simulink library "INT_CoETS_TrqCalc"  (R2016b)
settings: Solver=VariableStepAuto  StartTime=0.0  StopTime=10.0  RelTol=1e-3
settings Model: Creator=xuxingpei  LastModifiedBy=xuxingpei

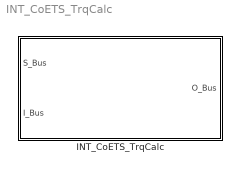
== system INT_CoETS_TrqCalc ==
  INT_CoETS_TrqCalc : Subsystem

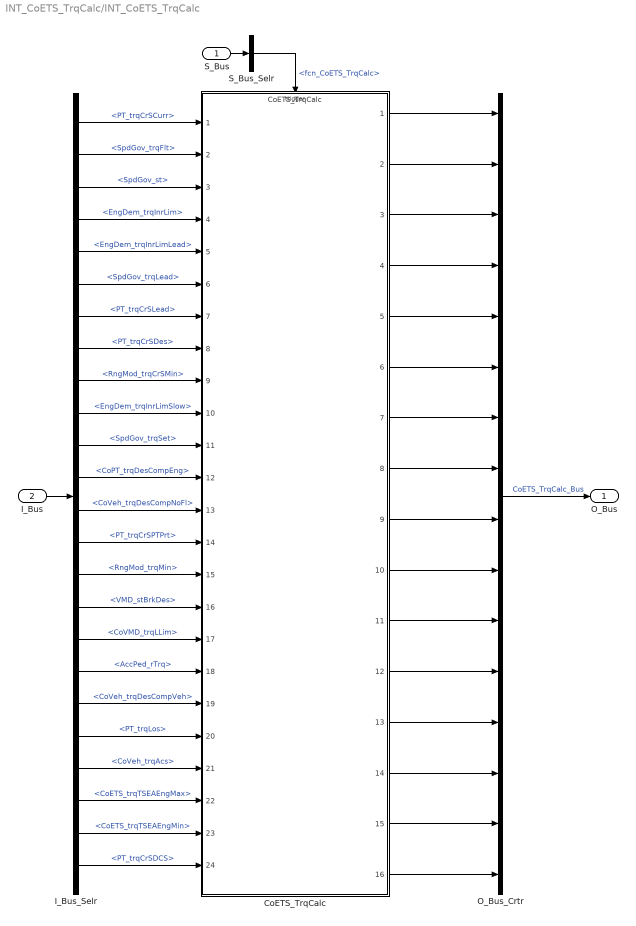
== system INT_CoETS_TrqCalc/INT_CoETS_TrqCalc ==
  S_Bus : Inport
  I_Bus : Inport  Port=2
  CoETS_TrqCalc : ModelReference  ModelNameDialog=CoETS_TrqCalc  SimulationMode=Normal  ModelReferenceVersion=1.18  TriggerPortName=function  TriggerPortTriggerType=function-call  TriggerPortStatesWhenEnabling=held
  I_Bus_Selr : BusSelector  OutputSignals=PT_trqCrSCurr,SpdGov_trqFlt,SpdGov_st,EngDem_trqInrLim,EngDem_trqInrLimLead,SpdGov_trqLead,PT_trqCrSLead,PT_trqCrSDes,RngMod_trqCrSMin,EngDem_trqInrLimSlow,SpdGov_trqSet,CoPT_trqDesCompEng,CoVeh_trqDesCompNoFl,PT_trqCrSPTPrt,RngMod_trqMin,VMD_stBrkDes,CoVMD_trqLLim,AccPed_rTrq,CoVeh_trqDesCompVeh,PT_trqLos,CoVeh_trqAcs,CoETS_trqTSEAEngMax,CoETS_trqTSEAEngMin,PT_trqCrSDCS
  O_Bus_Crtr : BusCreator  Inputs=16
  S_Bus_Selr : BusSelector  OutputSignals=fcn_CoETS_TrqCalc
  O_Bus : Outport
  wires:
  S_Bus_Selr/1 -> CoETS_TrqCalc/Trigger  "<fcn_CoETS_TrqCalc>"
  S_Bus/1 -> S_Bus_Selr/1
  I_Bus/1 -> I_Bus_Selr/1
  I_Bus_Selr/1 -> CoETS_TrqCalc/1  "<PT_trqCrSCurr>"
  I_Bus_Selr/2 -> CoETS_TrqCalc/2  "<SpdGov_trqFlt>"
  I_Bus_Selr/3 -> CoETS_TrqCalc/3  "<SpdGov_st>"
  I_Bus_Selr/4 -> CoETS_TrqCalc/4  "<EngDem_trqInrLim>"
  I_Bus_Selr/5 -> CoETS_TrqCalc/5  "<EngDem_trqInrLimLead>"
  I_Bus_Selr/6 -> CoETS_TrqCalc/6  "<SpdGov_trqLead>"
  I_Bus_Selr/7 -> CoETS_TrqCalc/7  "<PT_trqCrSLead>"
  I_Bus_Selr/8 -> CoETS_TrqCalc/8  "<PT_trqCrSDes>"
  I_Bus_Selr/9 -> CoETS_TrqCalc/9  "<RngMod_trqCrSMin>"
  I_Bus_Selr/10 -> CoETS_TrqCalc/10  "<EngDem_trqInrLimSlow>"
  I_Bus_Selr/11 -> CoETS_TrqCalc/11  "<SpdGov_trqSet>"
  I_Bus_Selr/12 -> CoETS_TrqCalc/12  "<CoPT_trqDesCompEng>"
  I_Bus_Selr/13 -> CoETS_TrqCalc/13  "<CoVeh_trqDesCompNoFl>"
  I_Bus_Selr/14 -> CoETS_TrqCalc/14  "<PT_trqCrSPTPrt>"
  I_Bus_Selr/15 -> CoETS_TrqCalc/15  "<RngMod_trqMin>"
  I_Bus_Selr/16 -> CoETS_TrqCalc/16  "<VMD_stBrkDes>"
  I_Bus_Selr/17 -> CoETS_TrqCalc/17  "<CoVMD_trqLLim>"
  I_Bus_Selr/18 -> CoETS_TrqCalc/18  "<AccPed_rTrq>"
  I_Bus_Selr/19 -> CoETS_TrqCalc/19  "<CoVeh_trqDesCompVeh>"
  I_Bus_Selr/20 -> CoETS_TrqCalc/20  "<PT_trqLos>"
  I_Bus_Selr/21 -> CoETS_TrqCalc/21  "<CoVeh_trqAcs>"
  I_Bus_Selr/22 -> CoETS_TrqCalc/22  "<CoETS_trqTSEAEngMax>"
  I_Bus_Selr/23 -> CoETS_TrqCalc/23  "<CoETS_trqTSEAEngMin>"
  I_Bus_Selr/24 -> CoETS_TrqCalc/24  "<PT_trqCrSDCS>"
  O_Bus_Crtr/1 -> O_Bus/1  "CoETS_TrqCalc_Bus"
  CoETS_TrqCalc/1 -> O_Bus_Crtr/1
  CoETS_TrqCalc/2 -> O_Bus_Crtr/2
  CoETS_TrqCalc/3 -> O_Bus_Crtr/3
  CoETS_TrqCalc/4 -> O_Bus_Crtr/4
  CoETS_TrqCalc/5 -> O_Bus_Crtr/5
  CoETS_TrqCalc/6 -> O_Bus_Crtr/6
  CoETS_TrqCalc/7 -> O_Bus_Crtr/7
  CoETS_TrqCalc/8 -> O_Bus_Crtr/8
  CoETS_TrqCalc/9 -> O_Bus_Crtr/9
  CoETS_TrqCalc/10 -> O_Bus_Crtr/10
  CoETS_TrqCalc/11 -> O_Bus_Crtr/11
  CoETS_TrqCalc/12 -> O_Bus_Crtr/12
  CoETS_TrqCalc/13 -> O_Bus_Crtr/13
  CoETS_TrqCalc/14 -> O_Bus_Crtr/14
  CoETS_TrqCalc/15 -> O_Bus_Crtr/15
  CoETS_TrqCalc/16 -> O_Bus_Crtr/16
